simulink model "GaussianFilter"  (Simulink 8.0)
settings: Solver=ode45  StartTime=0.0  StopTime=0.017  RelTol=1e-3
undefined symbols (not defined in the file): Fs, get, sided, Two
libraries: commfilt2 x4, commrandsrc2 x1, dspsnks4 x1, commutil2 x1
settings Model: Creator=Dimav  LastModifiedBy=Dimav

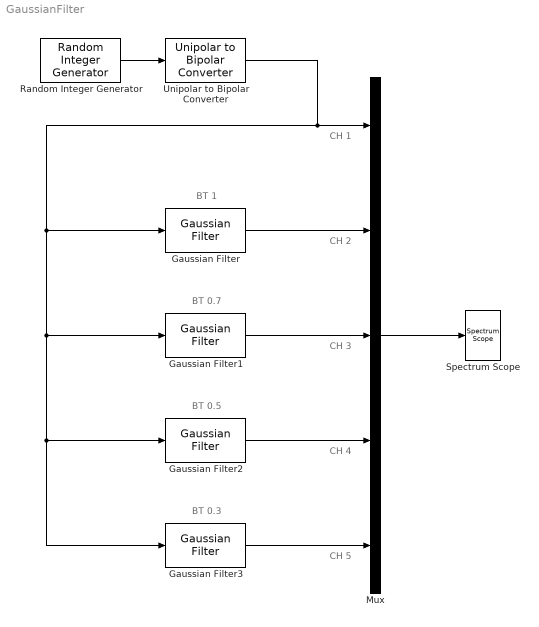
== system GaussianFilter ==
  note: BT 1
  note: CH 1
  note: CH 2
  note: CH 3
  note: CH 4
  note: CH 5
  note: BT 0.7
  note: BT 0.5
  note: BT 0.3
  Gaussian Filter : commfilt2/Gaussian Filter  N=8  BT=0.3  D=2  sampMode=Frame-based  normMode=Sum of coefficients  filterGain=1  checkCoeff=off  variableName=gaussFilt  launchFVT=off  roundingMode=Floor  overflowMode=off  InputProcessing=Columns as channels (frame based)
  Gaussian Filter1 : commfilt2/Gaussian Filter  N=8  BT=0.3  D=2  sampMode=Frame-based  normMode=Sum of coefficients  filterGain=1  checkCoeff=off  variableName=gaussFilt1  launchFVT=off  roundingMode=Floor  overflowMode=off  InputProcessing=Columns as channels (frame based)
  Gaussian Filter2 : commfilt2/Gaussian Filter  N=8  BT=0.3  D=2  sampMode=Frame-based  normMode=Sum of coefficients  filterGain=1  checkCoeff=off  variableName=gaussFilt2  launchFVT=off  roundingMode=Floor  overflowMode=off  InputProcessing=Columns as channels (frame based)
  Gaussian Filter3 : commfilt2/Gaussian Filter  N=8  BT=0.3  D=2  sampMode=Frame-based  normMode=Sum of coefficients  filterGain=1  checkCoeff=off  variableName=gaussFilt3  launchFVT=off  roundingMode=Floor  overflowMode=off  InputProcessing=Columns as channels (frame based)
  Mux : Mux  Inputs=5
  Random Integer Generator : commrandsrc2/Random Integer Generator  mul=2  seed=500  Ts=1/270000  frameBased=off  sampPerFrame=1  orient=off  outDataType=double
  Spectrum Scope : dspsnks4/Spectrum Scope  ScopeProperties=on  Domain=Frequency  HorizSpan=1  UseBuffer=on  BufferSize=128  Overlap=0  TreatMby1Signals=One channel  inpFftLenInherit=off  FFTlength=128  numAvg=2  DisplayProperties=off  AxisGrid=on  Memory=off  FrameNumber=on  AxisLegend=off  AxisZoom=off  OpenScopeAtSimStart=on  OpenScopeImmediately=off  FigPos=get(0,'defaultfigureposition')  AxisProperties=off  XUnits=Hertz  XRange=Two-sided ((-Fs/2...Fs/2])  XDisplay=0  InheritXIncr=on  XIncr=1.0  XLabel=Samples  XLimit=Auto  YUnits=Watts/Hertz  XMax=1  XMin=0  YLabel=Magnitude-squared, dB  LineProperties=off  wintypeSpecScope=Hann  RsSpecScope=50  betaSpecScope=5  winsampSpecScope=Periodic  XAxisParamsVer=6.9  isFrameUpgraded=on
      settings: YMin=-10  YMax=10
  Unipolar to Bipolar Converter : commutil2/Unipolar to Bipolar Converter  M=2  polarity=Positive  dataType=Inherit via internal rule
  wires:
  Random Integer Generator/1 -> Unipolar to Bipolar Converter/1
  Mux/1 -> Spectrum Scope/1
  Unipolar to Bipolar Converter/1 -> Gaussian Filter/1, Gaussian Filter3/1, Gaussian Filter2/1, Gaussian Filter1/1, Mux/1
  Gaussian Filter/1 -> Mux/2
  Gaussian Filter1/1 -> Mux/3
  Gaussian Filter2/1 -> Mux/4
  Gaussian Filter3/1 -> Mux/5
